simulink model "Part2_IV"  (R2023b)
settings: Solver=VariableStepAuto  StartTime=0.0  StopTime=1  RelTol=1e-3
libraries: simulink x1, commrandsrc3 x1
settings Model: Creator=henry  LastModifiedBy=henry

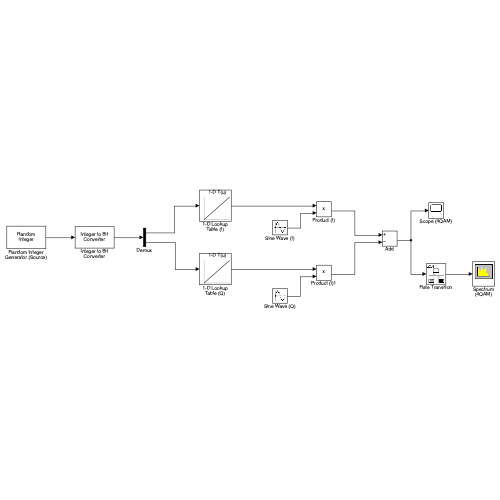
[thumbnail: Simulink's stored preview of the top-level diagram]
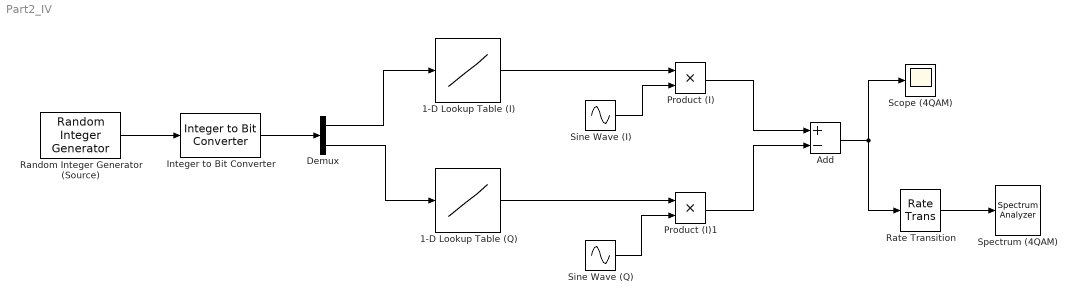
== system Part2_IV ==
  1-D Lookup Table (I) : Lookup_n-D  NumberOfTableDimensions=1  BreakpointsForDimension1=[0,1]  Table=[-sqrt(0.5),sqrt(0.5)]  InternalRulePriority=Speed  RndMeth=Simplest
  1-D Lookup Table (Q) : Lookup_n-D  NumberOfTableDimensions=1  BreakpointsForDimension1=[0,1]  Table=[-sqrt(0.5),sqrt(0.5)]  InternalRulePriority=Speed  RndMeth=Simplest
  Add : Sum  Inputs=+-
  Demux : Demux  Outputs=2
  Integer to Bit Converter : simulink/Logic and Bit Operations/Integer to Bit Converter  nbits=2  signedInputValues=Unsigned  bitOrder=MSB first  outDtype=Inherit via internal rule
  Product (I) : Product
  Product (I)1 : Product
  Random Integer Generator (Source) : commrandsrc3/Random Integer Generator  SetSize=4  SeedSource=Auto  Seed=0  SampleTime=0.001  SamplesPerFrame=1  OutputDataType=double  SimulateUsing=Interpreted execution
  Rate Transition : RateTransition  OutPortSampleTime=0.5e-4
  Scope (4QAM) : Scope
  Sine Wave (I) : Sin  SineType=Sample based  Samples=5000  SampleTime=1e-7  Offset=1250
  Sine Wave (Q) : Sin  SineType=Sample based  Samples=5000  SampleTime=1e-7
  Spectrum (4QAM) : SpectrumAnalyzer  WindowPosition=[80.000000,345.000000,800.000000,500.000000,]  ScopeFrameLocation=window  YLimits=[-60.74677965,15.3795234]
  wires:
  Random Integer Generator (Source)/1 -> Integer to Bit Converter/1
  Integer to Bit Converter/1 -> Demux/1
  Demux/1 -> 1-D Lookup Table (I)/1
  Demux/2 -> 1-D Lookup Table (Q)/1
  1-D Lookup Table (I)/1 -> Product (I)/1
  1-D Lookup Table (Q)/1 -> Product (I)1/1
  Sine Wave (I)/1 -> Product (I)/2
  Sine Wave (Q)/1 -> Product (I)1/2
  Product (I)/1 -> Add/1
  Product (I)1/1 -> Add/2
  Add/1 -> Scope (4QAM)/1, Rate Transition/1
  Rate Transition/1 -> Spectrum (4QAM)/1
